simulink model "Six_Step_Arduino_Simulink"  (R2020b)
settings: Solver=FixedStepDiscrete  StartTime=0.0  StopTime=10  RelTol=1e-3  EnableMultiTasking=on
libraries: arduinolib x10, simulink x1
settings Model: SILPILModeSetting=veronly  ExtModeTrigDuration=2  Creator=HP  LastModifiedBy=HP
settings OptimizationCC: EnhancedBackFolding=on  PassReuseOutputArgsAs=Individual arguments  ZeroExternalMemoryAtStartup=off  ZeroInternalMemoryAtStartup=off  MaxStackSize=64  OptimizeBlockOrder=speed  DifferentSizesBufferReuse=on  OptimizationCustomize=off  EfficientTunableParamExpr=on
settings DebuggingCC: ParameterTunabilityLossMsg=error
settings HardwareCC: ProdBitPerInt=16  ProdBitPerPointer=16  ProdBitPerSizeT=16  ProdBitPerPtrDiffT=16  ProdLargestAtomicFloat=None  ProdWordSize=8  ProdHWDeviceType=Atmel->AVR
settings SFSimCC: MATLABDynamicMemAlloc=off
settings RTWCC: Description=Embedded Coder  SystemTargetFile=ert.tlc  HardwareBoard=Arduino Mega 2560  TemplateMakefile=ert_default_tmf  Toolchain=Arduino AVR  BuildConfiguration=Faster Runs
settings CodeAppCC: ForceParamTrailComments=on  IgnoreCustomStorageClasses=off  OperatorAnnotations=on  SimulinkDataObjDesc=on  SFDataObjDesc=on  InsertBlockDesc=on
settings ERTTargetCC: SupportContinuousTime=on  SupportVariableSizeSignals=on  ExtModeStaticAllocSize=2048

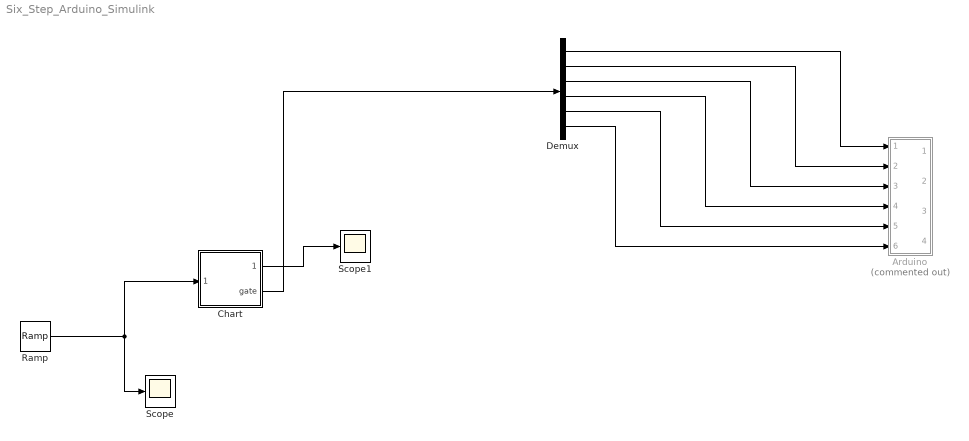
== system Six_Step_Arduino_Simulink ==
  Arduino : Subsystem  Commented=on
  Chart : Stateflow chart  TreatAsAtomicUnit=on
  Demux : Demux  Outputs=6
  Ramp : simulink/Sources/Ramp  slope=100  start=0  InitialOutput=500
  Scope : Scope
  Scope1 : Scope
  wires:
  Demux/1 -> Arduino/1(In1)
  Demux/2 -> Arduino/2(In2)
  Demux/3 -> Arduino/3(In3)
  Demux/4 -> Arduino/4(In4)
  Demux/5 -> Arduino/5(In5)
  Demux/6 -> Arduino/6(In6)
  Chart/2(gate) -> Demux/1
  Chart/1(ChartMode) -> Scope1/1
  Ramp/1 -> Scope/1, Chart/1(speed)

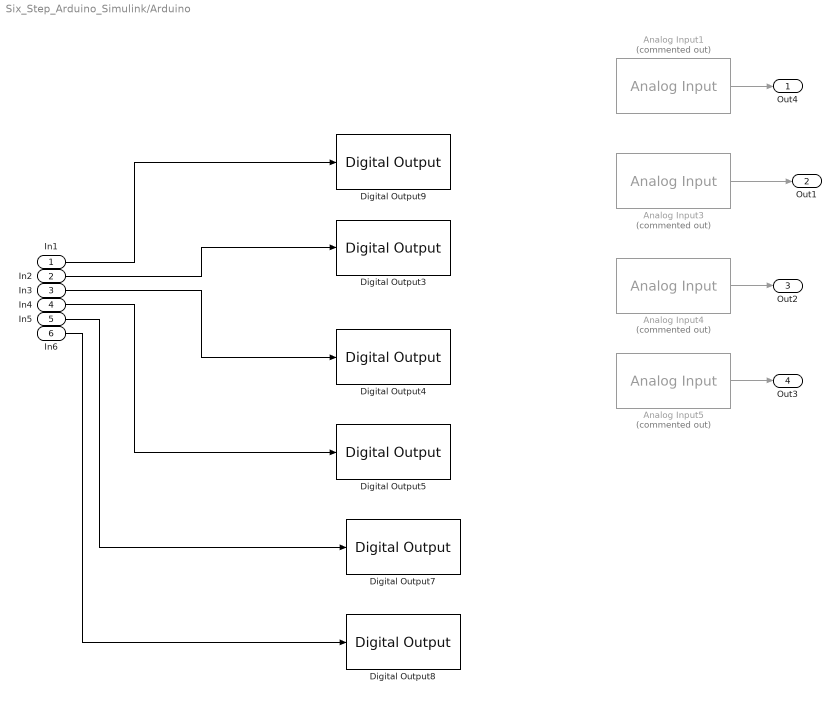
== system Six_Step_Arduino_Simulink/Arduino ==
  In1 : Inport
  In2 : Inport  Port=2
  In3 : Inport  Port=3
  In4 : Inport  Port=4
  In5 : Inport  Port=5
  In6 : Inport  Port=6
  Analog Input1 : arduinolib/Analog Input  Commented=on  pinNumber=0  ReadResultsOnly=off  ConversionTriggerSource=Software  ExternalTriggerType=uint32( 0 )  OutputDataType=uint16  EnableConversionCompleteNotify=off  EnableOuputStatus=off  SampleTime=-1  blockPlatform=arduino
  Analog Input3 : arduinolib/Analog Input  Commented=on  pinNumber=1  ReadResultsOnly=off  ConversionTriggerSource=Software  ExternalTriggerType=uint32( 0 )  OutputDataType=uint16  EnableConversionCompleteNotify=off  EnableOuputStatus=off  SampleTime=-1  blockPlatform=arduino
  Analog Input4 : arduinolib/Analog Input  Commented=on  pinNumber=2  ReadResultsOnly=off  ConversionTriggerSource=Software  ExternalTriggerType=uint32( 0 )  OutputDataType=uint16  EnableConversionCompleteNotify=off  EnableOuputStatus=off  SampleTime=-1  blockPlatform=arduino
  Analog Input5 : arduinolib/Analog Input  Commented=on  pinNumber=3  ReadResultsOnly=off  ConversionTriggerSource=Software  ExternalTriggerType=uint32( 0 )  OutputDataType=uint16  EnableConversionCompleteNotify=off  EnableOuputStatus=off  SampleTime=-1  blockPlatform=arduino
  Digital Output3 : arduinolib/Digital Output  pinNumber=3  Direction=output  blockPlatform=arduino
  Digital Output4 : arduinolib/Digital Output  pinNumber=4  Direction=output  blockPlatform=arduino
  Digital Output5 : arduinolib/Digital Output  pinNumber=5  Direction=output  blockPlatform=arduino
  Digital Output7 : arduinolib/Digital Output  pinNumber=6  Direction=output  blockPlatform=arduino
  Digital Output8 : arduinolib/Digital Output  pinNumber=7  Direction=output  blockPlatform=arduino
  Digital Output9 : arduinolib/Digital Output  pinNumber=2  Direction=output  blockPlatform=arduino
  Out4 : Outport
  Out1 : Outport  Port=2
  Out2 : Outport  Port=3
  Out3 : Outport  Port=4
  wires:
  In5/1 -> Digital Output7/1
  In6/1 -> Digital Output8/1
  In4/1 -> Digital Output5/1
  In1/1 -> Digital Output9/1
  In3/1 -> Digital Output4/1
  In2/1 -> Digital Output3/1
  Analog Input3/1 -> Out1/1
  Analog Input4/1 -> Out2/1
  Analog Input5/1 -> Out3/1
  Analog Input1/1 -> Out4/1

== stateflow chart Six_Step_Arduino_Simulink/Chart ==
  state State6
    entry:
    gate=[1 0 0 1 0 0]
  state State1
    entry:
    gate=[1 0 0 0 0 1]
  state State2
    entry:
    gate=[0 0 1 0 0 1]
  state State5
    entry:
    gate=[0 0 0 1 1 0]
  state State3
    entry:
    gate=[0 1 1 0 0 0]
  state State4
    entry:
    gate=[0 1 0 0 1 0]
  (default) -> State1
  State6 -> State1 : after(speed,usec)
  State5 -> State6 : after(speed,usec)
  State1 -> State2 : after(speed,usec)
  State4 -> State5 : after(speed,usec)
  State2 -> State3 : after(speed,usec)
  State3 -> State4 : after(speed,usec)
  data: ChartMode output Enum: ChartModeType; speed input; gate output
